simulink model "adc_demo"  (Simulink 8.3)
settings: Solver=VariableStepDiscrete  StartTime=0.0  StopTime=1  RelTol=1e-3
libraries: simulink_extras x1
settings Model: Creator=rcheng  LastModifiedBy=rodralez
settings OptimizationCC: ExpressionDepthLimit=2147483647  InitFltsAndDblsToZero=on
settings DebuggingCC: FcnCallInpInsideContextMsg=UseLocalSettings

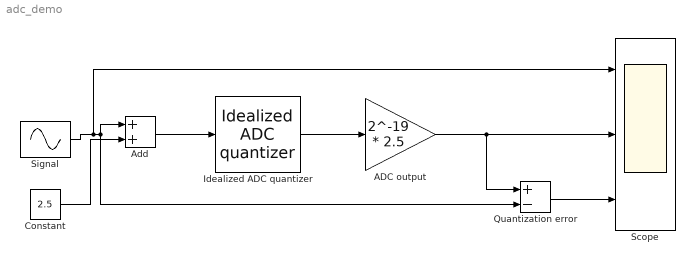
== system adc_demo ==
  ADC output : Gain  Gain=2^-19 * 2.5
  Add : Sum
  Constant : Constant  Value=2.5
  Idealized ADC quantizer : simulink_extras/Additional Discrete/Idealized ADC quantizer  NumberOfConverterBits=20  Vmin=0  Vmax=5  OutputDataType=int32  OutputNegativeValues=on
  Quantization error : Sum  Inputs=+-
  Scope : Scope  NumInputPorts=3
      settings: ShowLegends=on  TimeRange=0.5  YMin=-5~-5~-5  YMax=5~5~5
  Signal : Sin  Amplitude=2.5  Frequency=2*pi*100  SampleTime=1/10000
  wires:
  Quantization error/1 -> Scope/3
  Signal/1 -> Quantization error/2, Add/1, Scope/1
  Idealized ADC quantizer/1 -> ADC output/1
  Add/1 -> Idealized ADC quantizer/1
  Constant/1 -> Add/2
  ADC output/1 -> Quantization error/1, Scope/2
